simulink model "moto"  (R2026a)
settings: Solver=VariableStepAuto
InitFcn:
  | moto_init;
values from neighbouring files (symbols this model uses):
  nz = [0,0,1].'    [moto_init.m]
  p = motoParameters    [bikeSimToMotoParameters.m]    (also in moto_init.m = bikeSimToPrydeV2Parameters(bs,130/3.6); moto_trim_test.m = P{idx_vx}; steadyTurningTrimEqns.m = in3(41,:); steadyTurningTrimJac.m = in3(41,:))
  Scamber = rscrew('x',p_camber0)    [moto_init.m]
  Spitchr = rscrew('y',p_pitchr0)    [moto_init.m]
  Sx = pscrew('x')    [moto_init.m]
  Sy = pscrew('y')    [moto_init.m]
  Syaw = rscrew('z',p_yaw0)    [moto_init.m]
libraries: simulink_extras x3
settings Model: Creator=marti  LastModifiedBy=marti

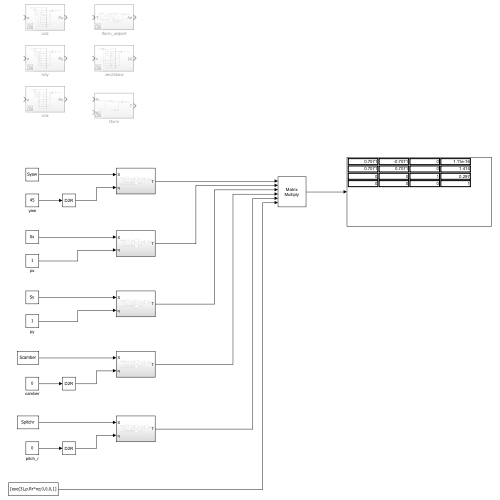
[thumbnail: Simulink's stored preview of the top-level diagram]
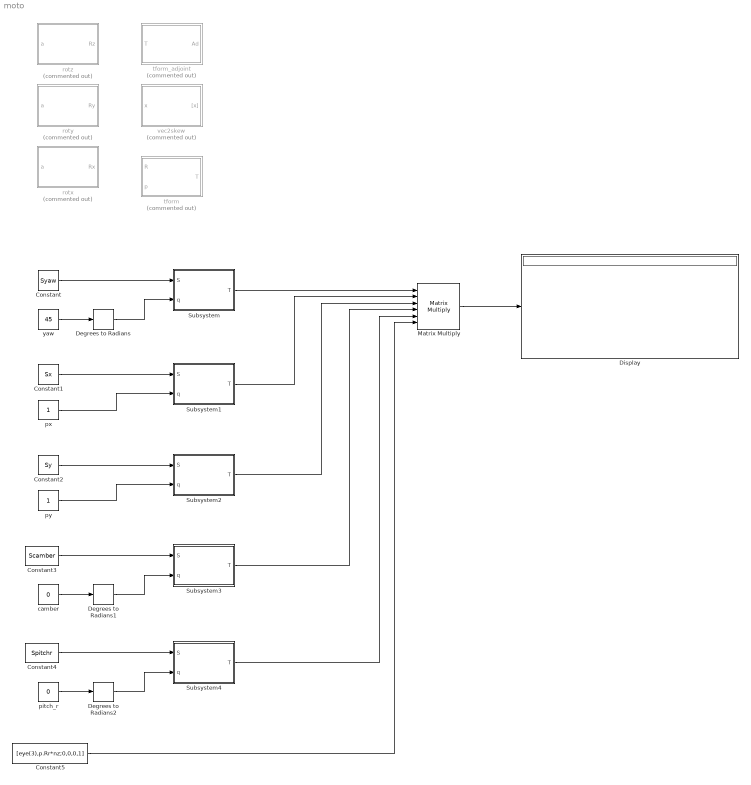
== system moto ==
  Constant : Constant  Value=Syaw
  Constant1 : Constant  Value=Sx
  Constant2 : Constant  Value=Sy
  Constant3 : Constant  Value=Scamber
  Constant4 : Constant  Value=Spitchr
  Constant5 : Constant  Value=[eye(3),p.Rr*nz;0,0,0,1]
  Degrees to Radians : simulink_extras/Transformations/Degrees to Radians
  Degrees to Radians1 : simulink_extras/Transformations/Degrees to Radians
  Degrees to Radians2 : simulink_extras/Transformations/Degrees to Radians
  Display : Display
  Matrix Multiply : Product  Inputs=6  Multiplication=Matrix(*)
  Subsystem : Subsystem
  Subsystem1 : Subsystem
  Subsystem2 : Subsystem
  Subsystem3 : Subsystem
  Subsystem4 : Subsystem
  camber : Constant  Value=0
  pitch_r : Constant  Value=0
  px : Constant
  py : Constant
  rotx : Subsystem  Commented=on
  roty : Subsystem  Commented=on
  rotz : Subsystem  Commented=on
  tform : Subsystem  Commented=on
  tform_adjoint : Subsystem  Commented=on
  vec2skew : Subsystem  Commented=on
  yaw : Constant  Value=45
  wires:
  yaw/1 -> Degrees to Radians/1
  Degrees to Radians/1 -> Subsystem/2(q)
  Constant/1 -> Subsystem/1(S)
  Constant1/1 -> Subsystem1/1(S)
  px/1 -> Subsystem1/2(q)
  Constant2/1 -> Subsystem2/1(S)
  py/1 -> Subsystem2/2(q)
  Constant3/1 -> Subsystem3/1(S)
  Degrees to Radians1/1 -> Subsystem3/2(q)
  camber/1 -> Degrees to Radians1/1
  pitch_r/1 -> Degrees to Radians2/1
  Degrees to Radians2/1 -> Subsystem4/2(q)
  Constant4/1 -> Subsystem4/1(S)
  Subsystem/1(T) -> Matrix Multiply/1
  Subsystem1/1(T) -> Matrix Multiply/2
  Subsystem2/1(T) -> Matrix Multiply/3
  Subsystem3/1(T) -> Matrix Multiply/4
  Subsystem4/1(T) -> Matrix Multiply/5
  Matrix Multiply/1 -> Display/1
  Constant5/1 -> Matrix Multiply/6

== system moto/Subsystem ==
  S : Inport
  q : Inport  Port=2
  Reshape : Reshape  OutputDimensionality=Column vector (2-D)
  Selector : Selector  InputPortWidth=6  IndexOptions=Index vector (dialog)  Indices=1:3  OutputSizes=1
  axisAngleToRotMat : Subsystem
  screwDistanceToPos : Subsystem
  tform : Subsystem
  T : Outport
  wires:
  S/1 -> Reshape/1
  Selector/1 -> axisAngleToRotMat/1(w)  "w"
  q/1 -> screwDistanceToPos/2(q), axisAngleToRotMat/2(q)
  axisAngleToRotMat/1(R) -> tform/1(R)
  tform/1(T) -> T/1
  screwDistanceToPos/1(p) -> tform/2(p)
  Reshape/1 -> screwDistanceToPos/1(S), Selector/1

== system moto/Subsystem1 ==
  S : Inport
  q : Inport  Port=2
  Reshape : Reshape  OutputDimensionality=Column vector (2-D)
  Selector : Selector  InputPortWidth=6  IndexOptions=Index vector (dialog)  Indices=1:3  OutputSizes=1
  axisAngleToRotMat : Subsystem
  screwDistanceToPos : Subsystem
  tform : Subsystem
  T : Outport
  wires:
  S/1 -> Reshape/1
  Selector/1 -> axisAngleToRotMat/1(w)  "w"
  q/1 -> screwDistanceToPos/2(q), axisAngleToRotMat/2(q)
  axisAngleToRotMat/1(R) -> tform/1(R)
  tform/1(T) -> T/1
  screwDistanceToPos/1(p) -> tform/2(p)
  Reshape/1 -> screwDistanceToPos/1(S), Selector/1

== system moto/Subsystem2 ==
  S : Inport
  q : Inport  Port=2
  Reshape : Reshape  OutputDimensionality=Column vector (2-D)
  Selector : Selector  InputPortWidth=6  IndexOptions=Index vector (dialog)  Indices=1:3  OutputSizes=1
  axisAngleToRotMat : Subsystem
  screwDistanceToPos : Subsystem
  tform : Subsystem
  T : Outport
  wires:
  S/1 -> Reshape/1
  Selector/1 -> axisAngleToRotMat/1(w)  "w"
  q/1 -> screwDistanceToPos/2(q), axisAngleToRotMat/2(q)
  axisAngleToRotMat/1(R) -> tform/1(R)
  tform/1(T) -> T/1
  screwDistanceToPos/1(p) -> tform/2(p)
  Reshape/1 -> screwDistanceToPos/1(S), Selector/1

== system moto/Subsystem3 ==
  S : Inport
  q : Inport  Port=2
  Reshape : Reshape  OutputDimensionality=Column vector (2-D)
  Selector : Selector  InputPortWidth=6  IndexOptions=Index vector (dialog)  Indices=1:3  OutputSizes=1
  axisAngleToRotMat : Subsystem
  screwDistanceToPos : Subsystem
  tform : Subsystem
  T : Outport
  wires:
  S/1 -> Reshape/1
  Selector/1 -> axisAngleToRotMat/1(w)  "w"
  q/1 -> screwDistanceToPos/2(q), axisAngleToRotMat/2(q)
  axisAngleToRotMat/1(R) -> tform/1(R)
  tform/1(T) -> T/1
  screwDistanceToPos/1(p) -> tform/2(p)
  Reshape/1 -> screwDistanceToPos/1(S), Selector/1

== system moto/Subsystem4 ==
  S : Inport
  q : Inport  Port=2
  Reshape : Reshape  OutputDimensionality=Column vector (2-D)
  Selector : Selector  InputPortWidth=6  IndexOptions=Index vector (dialog)  Indices=1:3  OutputSizes=1
  axisAngleToRotMat : Subsystem
  screwDistanceToPos : Subsystem
  tform : Subsystem
  T : Outport
  wires:
  S/1 -> Reshape/1
  Selector/1 -> axisAngleToRotMat/1(w)  "w"
  q/1 -> screwDistanceToPos/2(q), axisAngleToRotMat/2(q)
  axisAngleToRotMat/1(R) -> tform/1(R)
  tform/1(T) -> T/1
  screwDistanceToPos/1(p) -> tform/2(p)
  Reshape/1 -> screwDistanceToPos/1(S), Selector/1

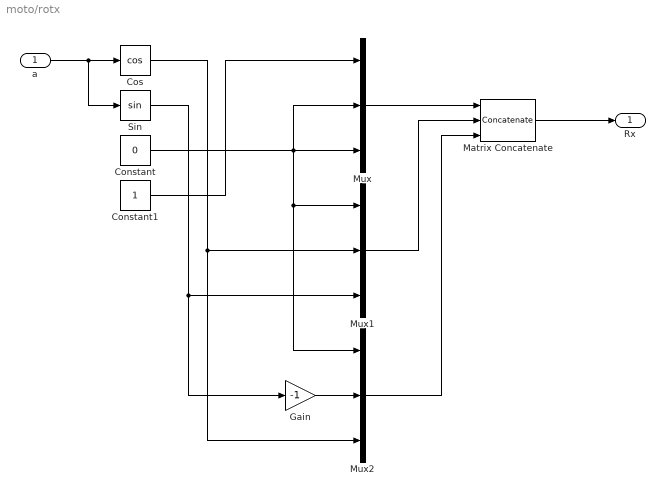
== system moto/rotx ==
  a : Inport
  Constant : Constant  Value=0
  Constant1 : Constant
  Cos : Trigonometry  Operator=cos
  Gain : Gain  Gain=-1
  Matrix Concatenate : Concatenate  NumInputs=3  Mode=Multidimensional array  ConcatenateDimension=2
  Mux : Mux  Inputs=3
  Mux1 : Mux  Inputs=3
  Mux2 : Mux  Inputs=3
  Sin : Trigonometry
  Rx : Outport
  wires:
  a/1 -> Sin/1, Cos/1
  Mux1/1 -> Matrix Concatenate/2
  Mux/1 -> Matrix Concatenate/1
  Mux2/1 -> Matrix Concatenate/3
  Matrix Concatenate/1 -> Rx/1
  Constant1/1 -> Mux/1
  Constant/1 -> Mux2/1, Mux1/1, Mux/3, Mux/2
  Gain/1 -> Mux2/2
  Sin/1 -> Mux1/3, Gain/1
  Cos/1 -> Mux2/3, Mux1/2

== system moto/roty ==
  a : Inport
  Constant : Constant  Value=0
  Constant1 : Constant
  Cos : Trigonometry  Operator=cos
  Gain : Gain  Gain=-1
  Matrix Concatenate : Concatenate  NumInputs=3  Mode=Multidimensional array  ConcatenateDimension=2
  Mux : Mux  Inputs=3
  Mux1 : Mux  Inputs=3
  Mux2 : Mux  Inputs=3
  Sin : Trigonometry
  Ry : Outport
  wires:
  a/1 -> Sin/1, Cos/1
  Mux1/1 -> Matrix Concatenate/2
  Mux/1 -> Matrix Concatenate/1
  Mux2/1 -> Matrix Concatenate/3
  Matrix Concatenate/1 -> Ry/1
  Gain/1 -> Mux/3
  Sin/1 -> Mux2/1, Gain/1
  Cos/1 -> Mux2/3, Mux/1
  Constant/1 -> Mux2/2, Mux1/3, Mux1/1, Mux/2
  Constant1/1 -> Mux1/2

== system moto/rotz ==
  a : Inport
  Constant : Constant  Value=0
  Constant1 : Constant
  Cos : Trigonometry  Operator=cos
  Gain : Gain  Gain=-1
  Matrix Concatenate : Concatenate  NumInputs=3  Mode=Multidimensional array  ConcatenateDimension=2
  Mux : Mux  Inputs=3
  Mux1 : Mux  Inputs=3
  Mux2 : Mux  Inputs=3
  Sin : Trigonometry
  Rz : Outport
  wires:
  Cos/1 -> Mux1/2, Mux/1
  Constant1/1 -> Mux2/3
  Sin/1 -> Mux/2, Gain/1
  a/1 -> Sin/1, Cos/1
  Constant/1 -> Mux/3, Mux2/2, Mux2/1, Mux1/3
  Gain/1 -> Mux1/1
  Mux1/1 -> Matrix Concatenate/2
  Mux/1 -> Matrix Concatenate/1
  Mux2/1 -> Matrix Concatenate/3
  Matrix Concatenate/1 -> Rz/1

== system moto/tform ==
  R : Inport
  p : Inport  Port=2
  Constant : Constant  Value=[0,0,0,1]
  Matrix Concatenate : Concatenate  Mode=Multidimensional array  ConcatenateDimension=2
  Matrix Concatenate2 : Concatenate  Mode=Multidimensional array
  Reshape : Reshape  OutputDimensionality=Row vector (2-D)
  T : Outport
  wires:
  p/1 -> Matrix Concatenate/2
  Constant/1 -> Reshape/1
  Matrix Concatenate/1 -> Matrix Concatenate2/1
  Matrix Concatenate2/1 -> T/1
  R/1 -> Matrix Concatenate/1
  Reshape/1 -> Matrix Concatenate2/2

== system moto/tform_adjoint ==
  T : Inport
  Constant : Constant  Value=zeros(3)
  Matrix Concatenate : Concatenate  Mode=Multidimensional array  ConcatenateDimension=2
  Matrix Concatenate1 : Concatenate  Mode=Multidimensional array  ConcatenateDimension=2
  Matrix Concatenate2 : Concatenate  Mode=Multidimensional array
  Matrix Multiply : Product  Multiplication=Matrix(*)
  Selector : Selector  NumberOfDimensions=2  InputPortWidth=3  IndexOptions=Index vector (dialog),Index vector (dialog)  Indices=1:3,1:3  OutputSizes=1,1
  Selector1 : Selector  NumberOfDimensions=2  InputPortWidth=3  IndexOptions=Index vector (dialog),Index vector (dialog)  Indices=1:3,4  OutputSizes=1,1
  vec2skew : Subsystem
  Ad : Outport
  wires:
  Selector1/1 -> vec2skew/1(x)
  Selector/1 -> Matrix Multiply/2, Matrix Concatenate1/2, Matrix Concatenate/1
  Constant/1 -> Matrix Concatenate/2
  vec2skew/1("[x]") -> Matrix Multiply/1
  Matrix Multiply/1 -> Matrix Concatenate1/1
  Matrix Concatenate1/1 -> Matrix Concatenate2/2
  Matrix Concatenate/1 -> Matrix Concatenate2/1
  Matrix Concatenate2/1 -> Ad/1
  T/1 -> Selector1/1, Selector/1

== system moto/vec2skew ==
  x : Inport
  Constant : Constant  Value=0
  Demux : Demux  Outputs=3
  Gain : Gain  Gain=-1
  Gain1 : Gain  Gain=-1
  Gain2 : Gain  Gain=-1
  Matrix Concatenate : Concatenate  NumInputs=3  Mode=Multidimensional array  ConcatenateDimension=2
  Mux : Mux  Inputs=3
  Mux1 : Mux  Inputs=3
  Mux2 : Mux  Inputs=3
  "[x]" : Outport
  wires:
  Mux1/1 -> Matrix Concatenate/2
  Mux/1 -> Matrix Concatenate/1
  Mux2/1 -> Matrix Concatenate/3
  Matrix Concatenate/1 -> "[x]"/1
  Gain/1 -> Mux/3
  Gain1/1 -> Mux1/1
  Gain2/1 -> Mux2/2
  Constant/1 -> Mux/1, Mux1/2, Mux2/3
  x/1 -> Demux/1
  Demux/3 -> Gain1/1, Mux/2  "z"
  Demux/2 -> Mux2/1, Gain/1  "y"
  Demux/1 -> Gain2/1, Mux1/3  "x"

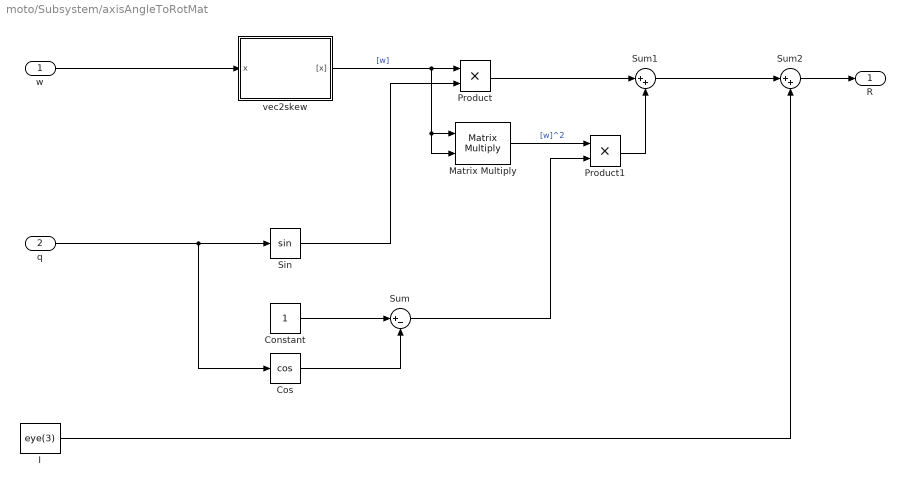
== system moto/Subsystem/axisAngleToRotMat ==
  w : Inport
  q : Inport  Port=2
  Constant : Constant
  Cos : Trigonometry  Operator=cos
  I : Constant  Value=eye(3)
  Matrix Multiply : Product  Multiplication=Matrix(*)
  Product : Product
  Product1 : Product
  Sin : Trigonometry
  Sum : Sum  Inputs=|+-
  Sum1 : Sum  Inputs=|++
  Sum2 : Sum  Inputs=|++
  vec2skew : Subsystem
  R : Outport
  wires:
  Cos/1 -> Sum/2
  Sum1/1 -> Sum2/1
  Sum/1 -> Product1/2
  Matrix Multiply/1 -> Product1/1  "[w]^2"
  Product1/1 -> Sum1/2
  Constant/1 -> Sum/1
  Product/1 -> Sum1/1
  I/1 -> Sum2/2
  vec2skew/1("[x]") -> Matrix Multiply/2, Matrix Multiply/1, Product/1  "[w]"
  Sin/1 -> Product/2
  q/1 -> Cos/1, Sin/1
  Sum2/1 -> R/1
  w/1 -> vec2skew/1(x)

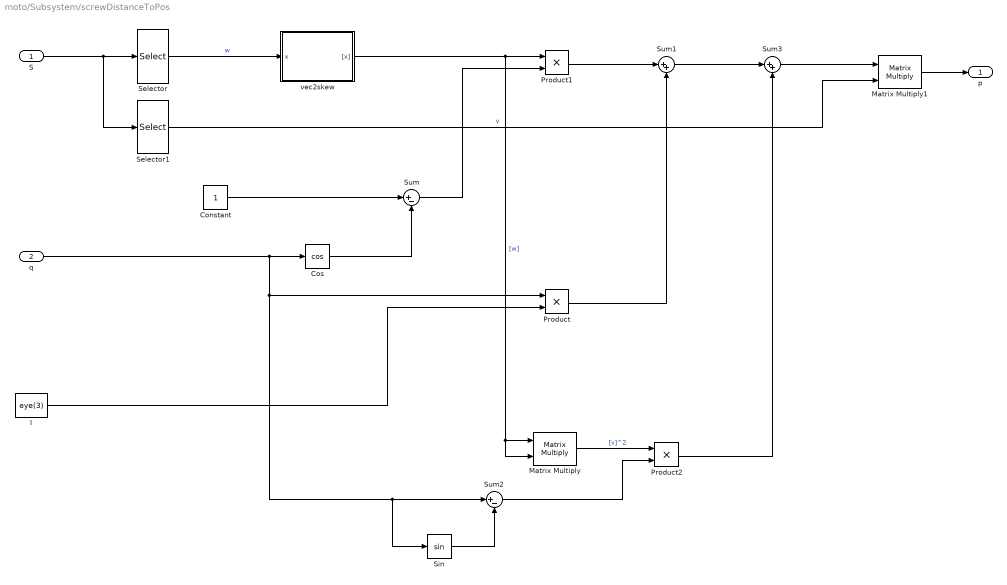
== system moto/Subsystem/screwDistanceToPos ==
  S : Inport
  q : Inport  Port=2
  Constant : Constant
  Cos : Trigonometry  Operator=cos
  I : Constant  Value=eye(3)
  Matrix Multiply : Product  Multiplication=Matrix(*)
  Matrix Multiply1 : Product  Multiplication=Matrix(*)
  Product : Product
  Product1 : Product
  Product2 : Product
  Selector : Selector  InputPortWidth=6  IndexOptions=Index vector (dialog)  Indices=1:3  OutputSizes=1
  Selector1 : Selector  InputPortWidth=6  IndexOptions=Index vector (dialog)  Indices=4:6  OutputSizes=1
  Sin : Trigonometry
  Sum : Sum  Inputs=|+-
  Sum1 : Sum  Inputs=|++
  Sum2 : Sum  Inputs=|+-
  Sum3 : Sum  Inputs=|++
  vec2skew : Subsystem
  p : Outport
  wires:
  Product/1 -> Sum1/2
  q/1 -> Cos/1, Product/1, Sin/1, Sum2/1
  Cos/1 -> Sum/2
  Constant/1 -> Sum/1
  vec2skew/1("[x]") -> Matrix Multiply/2, Matrix Multiply/1, Product1/1  "[w]"
  Sum2/1 -> Product2/2
  I/1 -> Product/2
  Product1/1 -> Sum1/1
  Sum/1 -> Product1/2
  Matrix Multiply/1 -> Product2/1  "[v]^2"
  Sum3/1 -> Matrix Multiply1/1
  Product2/1 -> Sum3/2
  Sin/1 -> Sum2/2
  Sum1/1 -> Sum3/1
  Selector1/1 -> Matrix Multiply1/2  "v"
  Matrix Multiply1/1 -> p/1
  Selector/1 -> vec2skew/1(x)  "w"
  S/1 -> Selector1/1, Selector/1

== system moto/Subsystem/tform ==
  R : Inport
  p : Inport  Port=2
  Constant : Constant  Value=[0,0,0,1]
  Matrix Concatenate : Concatenate  Mode=Multidimensional array  ConcatenateDimension=2
  Matrix Concatenate2 : Concatenate  Mode=Multidimensional array
  Reshape : Reshape  OutputDimensionality=Row vector (2-D)
  T : Outport
  wires:
  p/1 -> Matrix Concatenate/2
  Constant/1 -> Reshape/1
  Matrix Concatenate/1 -> Matrix Concatenate2/1
  Matrix Concatenate2/1 -> T/1
  R/1 -> Matrix Concatenate/1
  Reshape/1 -> Matrix Concatenate2/2

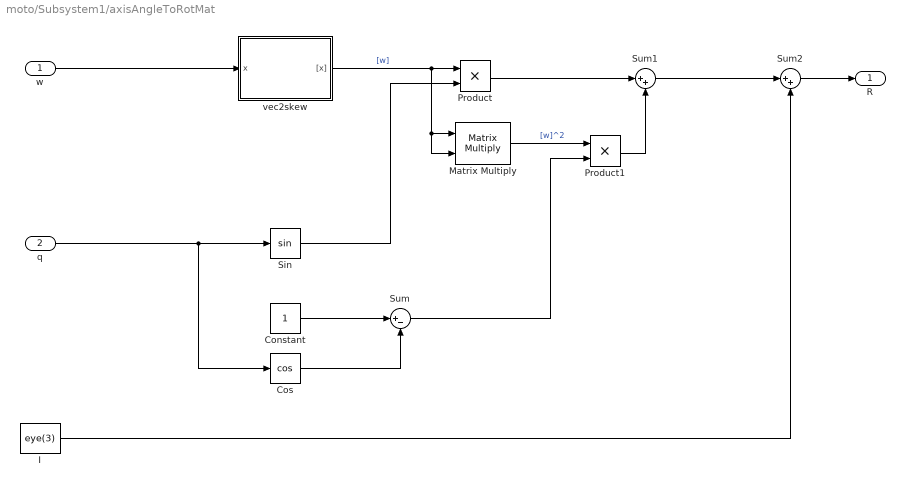
== system moto/Subsystem1/axisAngleToRotMat ==
  w : Inport
  q : Inport  Port=2
  Constant : Constant
  Cos : Trigonometry  Operator=cos
  I : Constant  Value=eye(3)
  Matrix Multiply : Product  Multiplication=Matrix(*)
  Product : Product
  Product1 : Product
  Sin : Trigonometry
  Sum : Sum  Inputs=|+-
  Sum1 : Sum  Inputs=|++
  Sum2 : Sum  Inputs=|++
  vec2skew : Subsystem
  R : Outport
  wires:
  Cos/1 -> Sum/2
  Sum1/1 -> Sum2/1
  Sum/1 -> Product1/2
  Matrix Multiply/1 -> Product1/1  "[w]^2"
  Product1/1 -> Sum1/2
  Constant/1 -> Sum/1
  Product/1 -> Sum1/1
  I/1 -> Sum2/2
  vec2skew/1("[x]") -> Matrix Multiply/2, Matrix Multiply/1, Product/1  "[w]"
  Sin/1 -> Product/2
  q/1 -> Cos/1, Sin/1
  Sum2/1 -> R/1
  w/1 -> vec2skew/1(x)

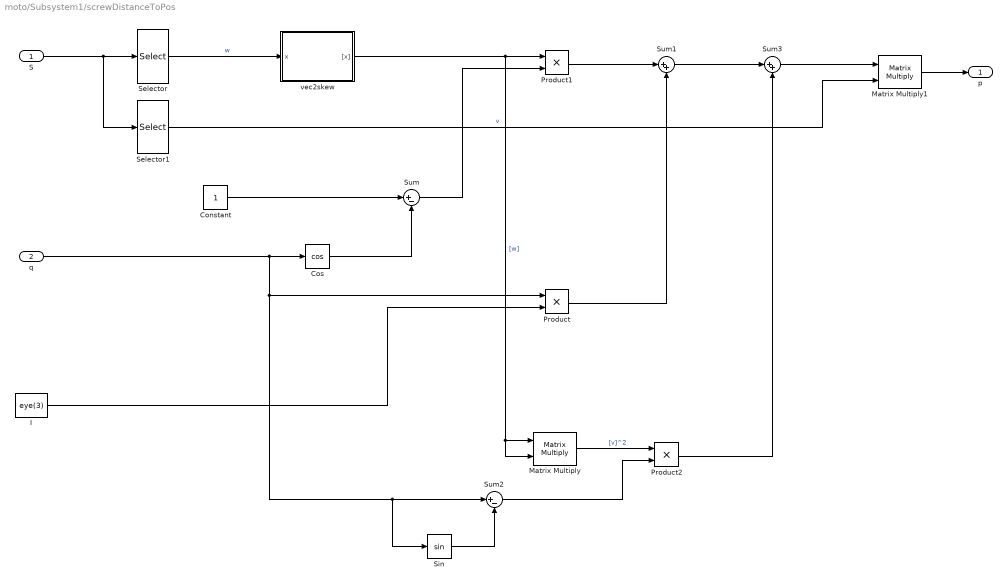
== system moto/Subsystem1/screwDistanceToPos ==
  S : Inport
  q : Inport  Port=2
  Constant : Constant
  Cos : Trigonometry  Operator=cos
  I : Constant  Value=eye(3)
  Matrix Multiply : Product  Multiplication=Matrix(*)
  Matrix Multiply1 : Product  Multiplication=Matrix(*)
  Product : Product
  Product1 : Product
  Product2 : Product
  Selector : Selector  InputPortWidth=6  IndexOptions=Index vector (dialog)  Indices=1:3  OutputSizes=1
  Selector1 : Selector  InputPortWidth=6  IndexOptions=Index vector (dialog)  Indices=4:6  OutputSizes=1
  Sin : Trigonometry
  Sum : Sum  Inputs=|+-
  Sum1 : Sum  Inputs=|++
  Sum2 : Sum  Inputs=|+-
  Sum3 : Sum  Inputs=|++
  vec2skew : Subsystem
  p : Outport
  wires:
  Product/1 -> Sum1/2
  q/1 -> Cos/1, Product/1, Sin/1, Sum2/1
  Cos/1 -> Sum/2
  Constant/1 -> Sum/1
  vec2skew/1("[x]") -> Matrix Multiply/2, Matrix Multiply/1, Product1/1  "[w]"
  Sum2/1 -> Product2/2
  I/1 -> Product/2
  Product1/1 -> Sum1/1
  Sum/1 -> Product1/2
  Matrix Multiply/1 -> Product2/1  "[v]^2"
  Sum3/1 -> Matrix Multiply1/1
  Product2/1 -> Sum3/2
  Sin/1 -> Sum2/2
  Sum1/1 -> Sum3/1
  Selector1/1 -> Matrix Multiply1/2  "v"
  Matrix Multiply1/1 -> p/1
  Selector/1 -> vec2skew/1(x)  "w"
  S/1 -> Selector1/1, Selector/1

== system moto/Subsystem1/tform ==
  R : Inport
  p : Inport  Port=2
  Constant : Constant  Value=[0,0,0,1]
  Matrix Concatenate : Concatenate  Mode=Multidimensional array  ConcatenateDimension=2
  Matrix Concatenate2 : Concatenate  Mode=Multidimensional array
  Reshape : Reshape  OutputDimensionality=Row vector (2-D)
  T : Outport
  wires:
  p/1 -> Matrix Concatenate/2
  Constant/1 -> Reshape/1
  Matrix Concatenate/1 -> Matrix Concatenate2/1
  Matrix Concatenate2/1 -> T/1
  R/1 -> Matrix Concatenate/1
  Reshape/1 -> Matrix Concatenate2/2

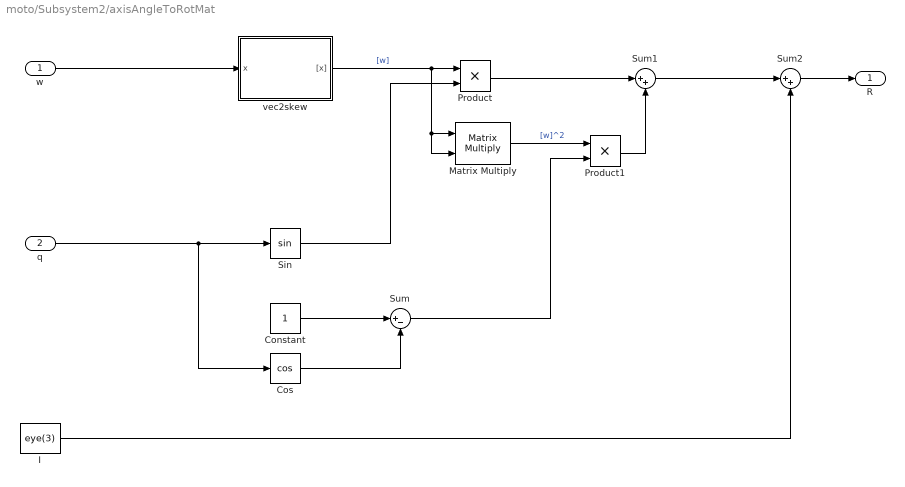
== system moto/Subsystem2/axisAngleToRotMat ==
  w : Inport
  q : Inport  Port=2
  Constant : Constant
  Cos : Trigonometry  Operator=cos
  I : Constant  Value=eye(3)
  Matrix Multiply : Product  Multiplication=Matrix(*)
  Product : Product
  Product1 : Product
  Sin : Trigonometry
  Sum : Sum  Inputs=|+-
  Sum1 : Sum  Inputs=|++
  Sum2 : Sum  Inputs=|++
  vec2skew : Subsystem
  R : Outport
  wires:
  Cos/1 -> Sum/2
  Sum1/1 -> Sum2/1
  Sum/1 -> Product1/2
  Matrix Multiply/1 -> Product1/1  "[w]^2"
  Product1/1 -> Sum1/2
  Constant/1 -> Sum/1
  Product/1 -> Sum1/1
  I/1 -> Sum2/2
  vec2skew/1("[x]") -> Matrix Multiply/2, Matrix Multiply/1, Product/1  "[w]"
  Sin/1 -> Product/2
  q/1 -> Cos/1, Sin/1
  Sum2/1 -> R/1
  w/1 -> vec2skew/1(x)

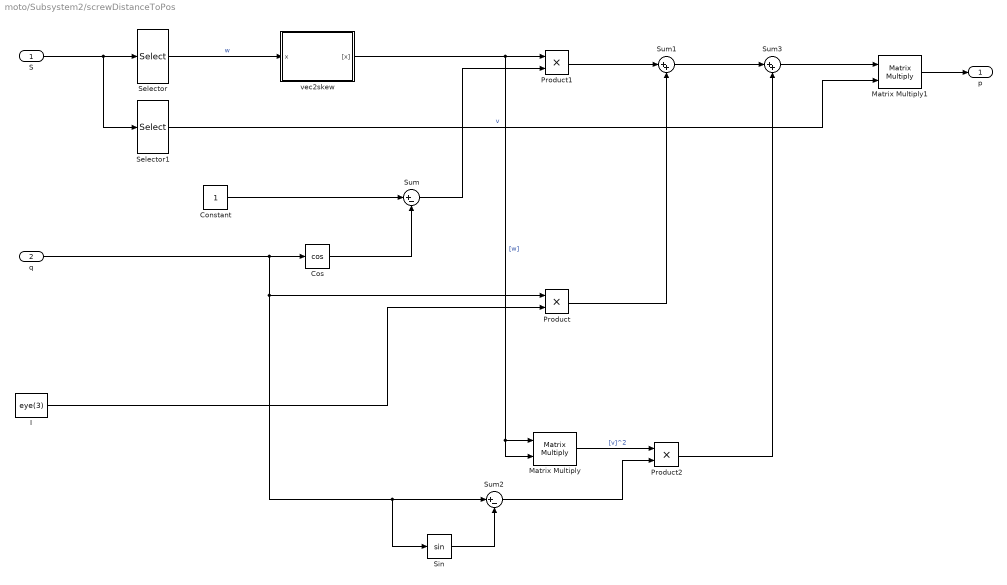
== system moto/Subsystem2/screwDistanceToPos ==
  S : Inport
  q : Inport  Port=2
  Constant : Constant
  Cos : Trigonometry  Operator=cos
  I : Constant  Value=eye(3)
  Matrix Multiply : Product  Multiplication=Matrix(*)
  Matrix Multiply1 : Product  Multiplication=Matrix(*)
  Product : Product
  Product1 : Product
  Product2 : Product
  Selector : Selector  InputPortWidth=6  IndexOptions=Index vector (dialog)  Indices=1:3  OutputSizes=1
  Selector1 : Selector  InputPortWidth=6  IndexOptions=Index vector (dialog)  Indices=4:6  OutputSizes=1
  Sin : Trigonometry
  Sum : Sum  Inputs=|+-
  Sum1 : Sum  Inputs=|++
  Sum2 : Sum  Inputs=|+-
  Sum3 : Sum  Inputs=|++
  vec2skew : Subsystem
  p : Outport
  wires:
  Product/1 -> Sum1/2
  q/1 -> Cos/1, Product/1, Sin/1, Sum2/1
  Cos/1 -> Sum/2
  Constant/1 -> Sum/1
  vec2skew/1("[x]") -> Matrix Multiply/2, Matrix Multiply/1, Product1/1  "[w]"
  Sum2/1 -> Product2/2
  I/1 -> Product/2
  Product1/1 -> Sum1/1
  Sum/1 -> Product1/2
  Matrix Multiply/1 -> Product2/1  "[v]^2"
  Sum3/1 -> Matrix Multiply1/1
  Product2/1 -> Sum3/2
  Sin/1 -> Sum2/2
  Sum1/1 -> Sum3/1
  Selector1/1 -> Matrix Multiply1/2  "v"
  Matrix Multiply1/1 -> p/1
  Selector/1 -> vec2skew/1(x)  "w"
  S/1 -> Selector1/1, Selector/1

== system moto/Subsystem2/tform ==
  R : Inport
  p : Inport  Port=2
  Constant : Constant  Value=[0,0,0,1]
  Matrix Concatenate : Concatenate  Mode=Multidimensional array  ConcatenateDimension=2
  Matrix Concatenate2 : Concatenate  Mode=Multidimensional array
  Reshape : Reshape  OutputDimensionality=Row vector (2-D)
  T : Outport
  wires:
  p/1 -> Matrix Concatenate/2
  Constant/1 -> Reshape/1
  Matrix Concatenate/1 -> Matrix Concatenate2/1
  Matrix Concatenate2/1 -> T/1
  R/1 -> Matrix Concatenate/1
  Reshape/1 -> Matrix Concatenate2/2

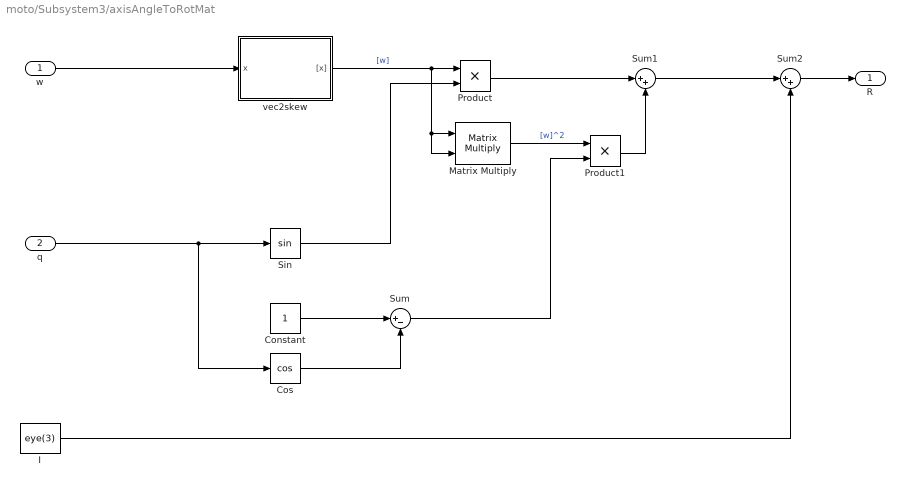
== system moto/Subsystem3/axisAngleToRotMat ==
  w : Inport
  q : Inport  Port=2
  Constant : Constant
  Cos : Trigonometry  Operator=cos
  I : Constant  Value=eye(3)
  Matrix Multiply : Product  Multiplication=Matrix(*)
  Product : Product
  Product1 : Product
  Sin : Trigonometry
  Sum : Sum  Inputs=|+-
  Sum1 : Sum  Inputs=|++
  Sum2 : Sum  Inputs=|++
  vec2skew : Subsystem
  R : Outport
  wires:
  Cos/1 -> Sum/2
  Sum1/1 -> Sum2/1
  Sum/1 -> Product1/2
  Matrix Multiply/1 -> Product1/1  "[w]^2"
  Product1/1 -> Sum1/2
  Constant/1 -> Sum/1
  Product/1 -> Sum1/1
  I/1 -> Sum2/2
  vec2skew/1("[x]") -> Matrix Multiply/2, Matrix Multiply/1, Product/1  "[w]"
  Sin/1 -> Product/2
  q/1 -> Cos/1, Sin/1
  Sum2/1 -> R/1
  w/1 -> vec2skew/1(x)

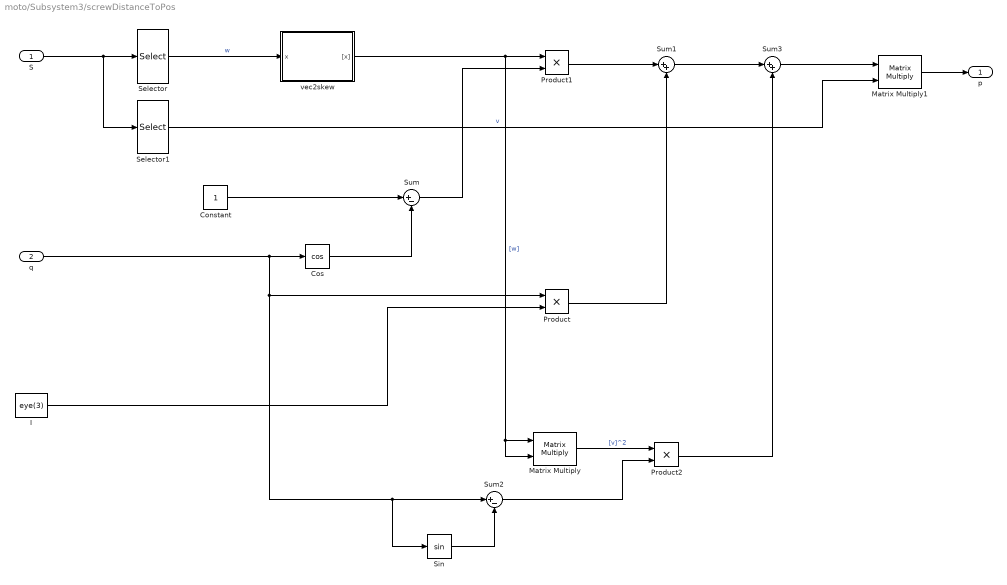
== system moto/Subsystem3/screwDistanceToPos ==
  S : Inport
  q : Inport  Port=2
  Constant : Constant
  Cos : Trigonometry  Operator=cos
  I : Constant  Value=eye(3)
  Matrix Multiply : Product  Multiplication=Matrix(*)
  Matrix Multiply1 : Product  Multiplication=Matrix(*)
  Product : Product
  Product1 : Product
  Product2 : Product
  Selector : Selector  InputPortWidth=6  IndexOptions=Index vector (dialog)  Indices=1:3  OutputSizes=1
  Selector1 : Selector  InputPortWidth=6  IndexOptions=Index vector (dialog)  Indices=4:6  OutputSizes=1
  Sin : Trigonometry
  Sum : Sum  Inputs=|+-
  Sum1 : Sum  Inputs=|++
  Sum2 : Sum  Inputs=|+-
  Sum3 : Sum  Inputs=|++
  vec2skew : Subsystem
  p : Outport
  wires:
  Product/1 -> Sum1/2
  q/1 -> Cos/1, Product/1, Sin/1, Sum2/1
  Cos/1 -> Sum/2
  Constant/1 -> Sum/1
  vec2skew/1("[x]") -> Matrix Multiply/2, Matrix Multiply/1, Product1/1  "[w]"
  Sum2/1 -> Product2/2
  I/1 -> Product/2
  Product1/1 -> Sum1/1
  Sum/1 -> Product1/2
  Matrix Multiply/1 -> Product2/1  "[v]^2"
  Sum3/1 -> Matrix Multiply1/1
  Product2/1 -> Sum3/2
  Sin/1 -> Sum2/2
  Sum1/1 -> Sum3/1
  Selector1/1 -> Matrix Multiply1/2  "v"
  Matrix Multiply1/1 -> p/1
  Selector/1 -> vec2skew/1(x)  "w"
  S/1 -> Selector1/1, Selector/1

== system moto/Subsystem3/tform ==
  R : Inport
  p : Inport  Port=2
  Constant : Constant  Value=[0,0,0,1]
  Matrix Concatenate : Concatenate  Mode=Multidimensional array  ConcatenateDimension=2
  Matrix Concatenate2 : Concatenate  Mode=Multidimensional array
  Reshape : Reshape  OutputDimensionality=Row vector (2-D)
  T : Outport
  wires:
  p/1 -> Matrix Concatenate/2
  Constant/1 -> Reshape/1
  Matrix Concatenate/1 -> Matrix Concatenate2/1
  Matrix Concatenate2/1 -> T/1
  R/1 -> Matrix Concatenate/1
  Reshape/1 -> Matrix Concatenate2/2

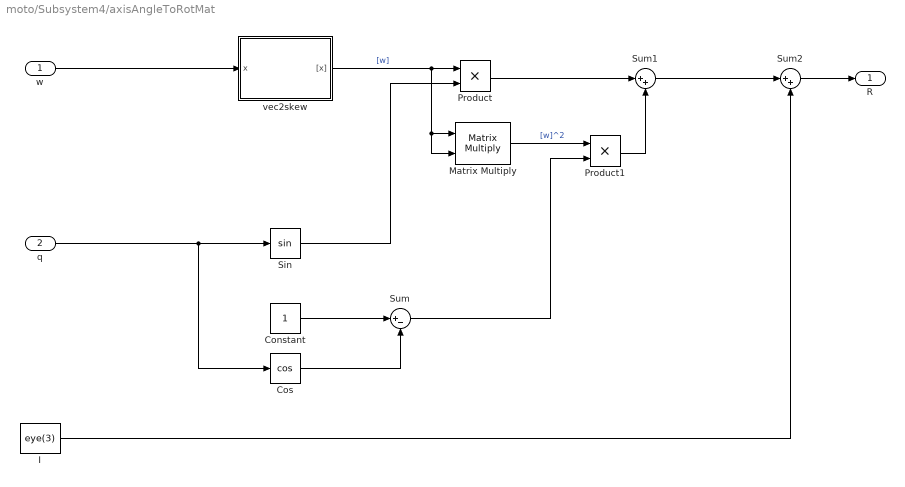
== system moto/Subsystem4/axisAngleToRotMat ==
  w : Inport
  q : Inport  Port=2
  Constant : Constant
  Cos : Trigonometry  Operator=cos
  I : Constant  Value=eye(3)
  Matrix Multiply : Product  Multiplication=Matrix(*)
  Product : Product
  Product1 : Product
  Sin : Trigonometry
  Sum : Sum  Inputs=|+-
  Sum1 : Sum  Inputs=|++
  Sum2 : Sum  Inputs=|++
  vec2skew : Subsystem
  R : Outport
  wires:
  Cos/1 -> Sum/2
  Sum1/1 -> Sum2/1
  Sum/1 -> Product1/2
  Matrix Multiply/1 -> Product1/1  "[w]^2"
  Product1/1 -> Sum1/2
  Constant/1 -> Sum/1
  Product/1 -> Sum1/1
  I/1 -> Sum2/2
  vec2skew/1("[x]") -> Matrix Multiply/2, Matrix Multiply/1, Product/1  "[w]"
  Sin/1 -> Product/2
  q/1 -> Cos/1, Sin/1
  Sum2/1 -> R/1
  w/1 -> vec2skew/1(x)

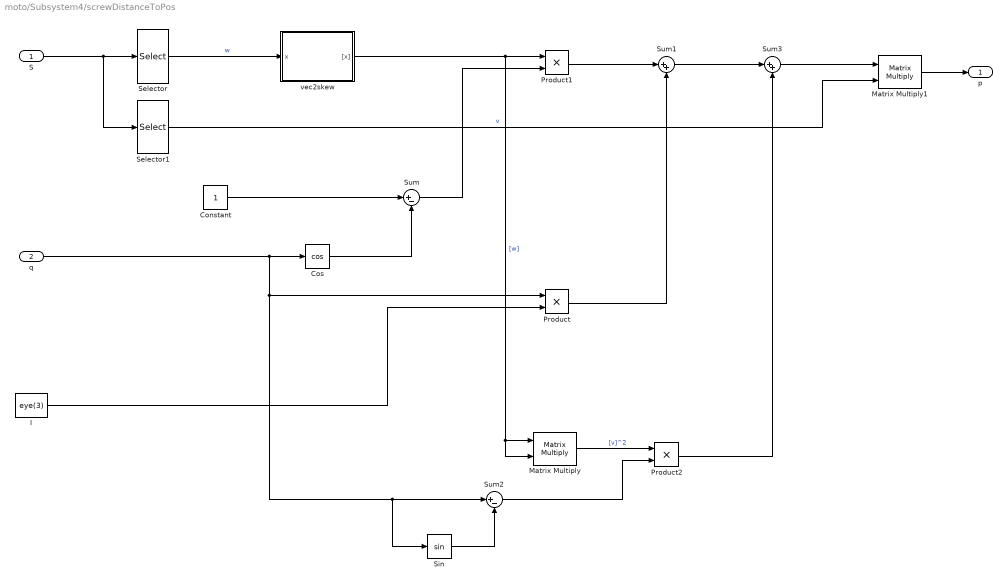
== system moto/Subsystem4/screwDistanceToPos ==
  S : Inport
  q : Inport  Port=2
  Constant : Constant
  Cos : Trigonometry  Operator=cos
  I : Constant  Value=eye(3)
  Matrix Multiply : Product  Multiplication=Matrix(*)
  Matrix Multiply1 : Product  Multiplication=Matrix(*)
  Product : Product
  Product1 : Product
  Product2 : Product
  Selector : Selector  InputPortWidth=6  IndexOptions=Index vector (dialog)  Indices=1:3  OutputSizes=1
  Selector1 : Selector  InputPortWidth=6  IndexOptions=Index vector (dialog)  Indices=4:6  OutputSizes=1
  Sin : Trigonometry
  Sum : Sum  Inputs=|+-
  Sum1 : Sum  Inputs=|++
  Sum2 : Sum  Inputs=|+-
  Sum3 : Sum  Inputs=|++
  vec2skew : Subsystem
  p : Outport
  wires:
  Product/1 -> Sum1/2
  q/1 -> Cos/1, Product/1, Sin/1, Sum2/1
  Cos/1 -> Sum/2
  Constant/1 -> Sum/1
  vec2skew/1("[x]") -> Matrix Multiply/2, Matrix Multiply/1, Product1/1  "[w]"
  Sum2/1 -> Product2/2
  I/1 -> Product/2
  Product1/1 -> Sum1/1
  Sum/1 -> Product1/2
  Matrix Multiply/1 -> Product2/1  "[v]^2"
  Sum3/1 -> Matrix Multiply1/1
  Product2/1 -> Sum3/2
  Sin/1 -> Sum2/2
  Sum1/1 -> Sum3/1
  Selector1/1 -> Matrix Multiply1/2  "v"
  Matrix Multiply1/1 -> p/1
  Selector/1 -> vec2skew/1(x)  "w"
  S/1 -> Selector1/1, Selector/1

== system moto/Subsystem4/tform ==
  R : Inport
  p : Inport  Port=2
  Constant : Constant  Value=[0,0,0,1]
  Matrix Concatenate : Concatenate  Mode=Multidimensional array  ConcatenateDimension=2
  Matrix Concatenate2 : Concatenate  Mode=Multidimensional array
  Reshape : Reshape  OutputDimensionality=Row vector (2-D)
  T : Outport
  wires:
  p/1 -> Matrix Concatenate/2
  Constant/1 -> Reshape/1
  Matrix Concatenate/1 -> Matrix Concatenate2/1
  Matrix Concatenate2/1 -> T/1
  R/1 -> Matrix Concatenate/1
  Reshape/1 -> Matrix Concatenate2/2

== system moto/tform_adjoint/vec2skew ==
  x : Inport
  Constant : Constant  Value=0
  Demux : Demux  Outputs=3
  Gain : Gain  Gain=-1
  Gain1 : Gain  Gain=-1
  Gain2 : Gain  Gain=-1
  Matrix Concatenate : Concatenate  NumInputs=3  Mode=Multidimensional array  ConcatenateDimension=2
  Mux : Mux  Inputs=3
  Mux1 : Mux  Inputs=3
  Mux2 : Mux  Inputs=3
  "[x]" : Outport
  wires:
  Mux1/1 -> Matrix Concatenate/2
  Mux/1 -> Matrix Concatenate/1
  Mux2/1 -> Matrix Concatenate/3
  Matrix Concatenate/1 -> "[x]"/1
  Gain/1 -> Mux/3
  Gain1/1 -> Mux1/1
  Gain2/1 -> Mux2/2
  Constant/1 -> Mux/1, Mux1/2, Mux2/3
  x/1 -> Demux/1
  Demux/3 -> Gain1/1, Mux/2  "z"
  Demux/2 -> Mux2/1, Gain/1  "y"
  Demux/1 -> Gain2/1, Mux1/3  "x"

== system moto/Subsystem/axisAngleToRotMat/vec2skew ==
  x : Inport
  Constant : Constant  Value=0
  Demux : Demux  Outputs=3
  Gain : Gain  Gain=-1
  Gain1 : Gain  Gain=-1
  Gain2 : Gain  Gain=-1
  Matrix Concatenate : Concatenate  NumInputs=3  Mode=Multidimensional array  ConcatenateDimension=2
  Mux : Mux  Inputs=3
  Mux1 : Mux  Inputs=3
  Mux2 : Mux  Inputs=3
  "[x]" : Outport
  wires:
  Mux1/1 -> Matrix Concatenate/2
  Mux/1 -> Matrix Concatenate/1
  Mux2/1 -> Matrix Concatenate/3
  Matrix Concatenate/1 -> "[x]"/1
  Gain/1 -> Mux/3
  Gain1/1 -> Mux1/1
  Gain2/1 -> Mux2/2
  Constant/1 -> Mux/1, Mux1/2, Mux2/3
  x/1 -> Demux/1
  Demux/3 -> Gain1/1, Mux/2  "z"
  Demux/2 -> Mux2/1, Gain/1  "y"
  Demux/1 -> Gain2/1, Mux1/3  "x"

== system moto/Subsystem/screwDistanceToPos/vec2skew ==
  x : Inport
  Constant : Constant  Value=0
  Demux : Demux  Outputs=3
  Gain : Gain  Gain=-1
  Gain1 : Gain  Gain=-1
  Gain2 : Gain  Gain=-1
  Matrix Concatenate : Concatenate  NumInputs=3  Mode=Multidimensional array  ConcatenateDimension=2
  Mux : Mux  Inputs=3
  Mux1 : Mux  Inputs=3
  Mux2 : Mux  Inputs=3
  "[x]" : Outport
  wires:
  Mux1/1 -> Matrix Concatenate/2
  Mux/1 -> Matrix Concatenate/1
  Mux2/1 -> Matrix Concatenate/3
  Matrix Concatenate/1 -> "[x]"/1
  Gain/1 -> Mux/3
  Gain1/1 -> Mux1/1
  Gain2/1 -> Mux2/2
  Constant/1 -> Mux/1, Mux1/2, Mux2/3
  x/1 -> Demux/1
  Demux/3 -> Gain1/1, Mux/2  "z"
  Demux/2 -> Mux2/1, Gain/1  "y"
  Demux/1 -> Gain2/1, Mux1/3  "x"

== system moto/Subsystem1/axisAngleToRotMat/vec2skew ==
  x : Inport
  Constant : Constant  Value=0
  Demux : Demux  Outputs=3
  Gain : Gain  Gain=-1
  Gain1 : Gain  Gain=-1
  Gain2 : Gain  Gain=-1
  Matrix Concatenate : Concatenate  NumInputs=3  Mode=Multidimensional array  ConcatenateDimension=2
  Mux : Mux  Inputs=3
  Mux1 : Mux  Inputs=3
  Mux2 : Mux  Inputs=3
  "[x]" : Outport
  wires:
  Mux1/1 -> Matrix Concatenate/2
  Mux/1 -> Matrix Concatenate/1
  Mux2/1 -> Matrix Concatenate/3
  Matrix Concatenate/1 -> "[x]"/1
  Gain/1 -> Mux/3
  Gain1/1 -> Mux1/1
  Gain2/1 -> Mux2/2
  Constant/1 -> Mux/1, Mux1/2, Mux2/3
  x/1 -> Demux/1
  Demux/3 -> Gain1/1, Mux/2  "z"
  Demux/2 -> Mux2/1, Gain/1  "y"
  Demux/1 -> Gain2/1, Mux1/3  "x"

== system moto/Subsystem1/screwDistanceToPos/vec2skew ==
  x : Inport
  Constant : Constant  Value=0
  Demux : Demux  Outputs=3
  Gain : Gain  Gain=-1
  Gain1 : Gain  Gain=-1
  Gain2 : Gain  Gain=-1
  Matrix Concatenate : Concatenate  NumInputs=3  Mode=Multidimensional array  ConcatenateDimension=2
  Mux : Mux  Inputs=3
  Mux1 : Mux  Inputs=3
  Mux2 : Mux  Inputs=3
  "[x]" : Outport
  wires:
  Mux1/1 -> Matrix Concatenate/2
  Mux/1 -> Matrix Concatenate/1
  Mux2/1 -> Matrix Concatenate/3
  Matrix Concatenate/1 -> "[x]"/1
  Gain/1 -> Mux/3
  Gain1/1 -> Mux1/1
  Gain2/1 -> Mux2/2
  Constant/1 -> Mux/1, Mux1/2, Mux2/3
  x/1 -> Demux/1
  Demux/3 -> Gain1/1, Mux/2  "z"
  Demux/2 -> Mux2/1, Gain/1  "y"
  Demux/1 -> Gain2/1, Mux1/3  "x"

== system moto/Subsystem2/axisAngleToRotMat/vec2skew ==
  x : Inport
  Constant : Constant  Value=0
  Demux : Demux  Outputs=3
  Gain : Gain  Gain=-1
  Gain1 : Gain  Gain=-1
  Gain2 : Gain  Gain=-1
  Matrix Concatenate : Concatenate  NumInputs=3  Mode=Multidimensional array  ConcatenateDimension=2
  Mux : Mux  Inputs=3
  Mux1 : Mux  Inputs=3
  Mux2 : Mux  Inputs=3
  "[x]" : Outport
  wires:
  Mux1/1 -> Matrix Concatenate/2
  Mux/1 -> Matrix Concatenate/1
  Mux2/1 -> Matrix Concatenate/3
  Matrix Concatenate/1 -> "[x]"/1
  Gain/1 -> Mux/3
  Gain1/1 -> Mux1/1
  Gain2/1 -> Mux2/2
  Constant/1 -> Mux/1, Mux1/2, Mux2/3
  x/1 -> Demux/1
  Demux/3 -> Gain1/1, Mux/2  "z"
  Demux/2 -> Mux2/1, Gain/1  "y"
  Demux/1 -> Gain2/1, Mux1/3  "x"

== system moto/Subsystem2/screwDistanceToPos/vec2skew ==
  x : Inport
  Constant : Constant  Value=0
  Demux : Demux  Outputs=3
  Gain : Gain  Gain=-1
  Gain1 : Gain  Gain=-1
  Gain2 : Gain  Gain=-1
  Matrix Concatenate : Concatenate  NumInputs=3  Mode=Multidimensional array  ConcatenateDimension=2
  Mux : Mux  Inputs=3
  Mux1 : Mux  Inputs=3
  Mux2 : Mux  Inputs=3
  "[x]" : Outport
  wires:
  Mux1/1 -> Matrix Concatenate/2
  Mux/1 -> Matrix Concatenate/1
  Mux2/1 -> Matrix Concatenate/3
  Matrix Concatenate/1 -> "[x]"/1
  Gain/1 -> Mux/3
  Gain1/1 -> Mux1/1
  Gain2/1 -> Mux2/2
  Constant/1 -> Mux/1, Mux1/2, Mux2/3
  x/1 -> Demux/1
  Demux/3 -> Gain1/1, Mux/2  "z"
  Demux/2 -> Mux2/1, Gain/1  "y"
  Demux/1 -> Gain2/1, Mux1/3  "x"

== system moto/Subsystem3/axisAngleToRotMat/vec2skew ==
  x : Inport
  Constant : Constant  Value=0
  Demux : Demux  Outputs=3
  Gain : Gain  Gain=-1
  Gain1 : Gain  Gain=-1
  Gain2 : Gain  Gain=-1
  Matrix Concatenate : Concatenate  NumInputs=3  Mode=Multidimensional array  ConcatenateDimension=2
  Mux : Mux  Inputs=3
  Mux1 : Mux  Inputs=3
  Mux2 : Mux  Inputs=3
  "[x]" : Outport
  wires:
  Mux1/1 -> Matrix Concatenate/2
  Mux/1 -> Matrix Concatenate/1
  Mux2/1 -> Matrix Concatenate/3
  Matrix Concatenate/1 -> "[x]"/1
  Gain/1 -> Mux/3
  Gain1/1 -> Mux1/1
  Gain2/1 -> Mux2/2
  Constant/1 -> Mux/1, Mux1/2, Mux2/3
  x/1 -> Demux/1
  Demux/3 -> Gain1/1, Mux/2  "z"
  Demux/2 -> Mux2/1, Gain/1  "y"
  Demux/1 -> Gain2/1, Mux1/3  "x"

== system moto/Subsystem3/screwDistanceToPos/vec2skew ==
  x : Inport
  Constant : Constant  Value=0
  Demux : Demux  Outputs=3
  Gain : Gain  Gain=-1
  Gain1 : Gain  Gain=-1
  Gain2 : Gain  Gain=-1
  Matrix Concatenate : Concatenate  NumInputs=3  Mode=Multidimensional array  ConcatenateDimension=2
  Mux : Mux  Inputs=3
  Mux1 : Mux  Inputs=3
  Mux2 : Mux  Inputs=3
  "[x]" : Outport
  wires:
  Mux1/1 -> Matrix Concatenate/2
  Mux/1 -> Matrix Concatenate/1
  Mux2/1 -> Matrix Concatenate/3
  Matrix Concatenate/1 -> "[x]"/1
  Gain/1 -> Mux/3
  Gain1/1 -> Mux1/1
  Gain2/1 -> Mux2/2
  Constant/1 -> Mux/1, Mux1/2, Mux2/3
  x/1 -> Demux/1
  Demux/3 -> Gain1/1, Mux/2  "z"
  Demux/2 -> Mux2/1, Gain/1  "y"
  Demux/1 -> Gain2/1, Mux1/3  "x"

== system moto/Subsystem4/axisAngleToRotMat/vec2skew ==
  x : Inport
  Constant : Constant  Value=0
  Demux : Demux  Outputs=3
  Gain : Gain  Gain=-1
  Gain1 : Gain  Gain=-1
  Gain2 : Gain  Gain=-1
  Matrix Concatenate : Concatenate  NumInputs=3  Mode=Multidimensional array  ConcatenateDimension=2
  Mux : Mux  Inputs=3
  Mux1 : Mux  Inputs=3
  Mux2 : Mux  Inputs=3
  "[x]" : Outport
  wires:
  Mux1/1 -> Matrix Concatenate/2
  Mux/1 -> Matrix Concatenate/1
  Mux2/1 -> Matrix Concatenate/3
  Matrix Concatenate/1 -> "[x]"/1
  Gain/1 -> Mux/3
  Gain1/1 -> Mux1/1
  Gain2/1 -> Mux2/2
  Constant/1 -> Mux/1, Mux1/2, Mux2/3
  x/1 -> Demux/1
  Demux/3 -> Gain1/1, Mux/2  "z"
  Demux/2 -> Mux2/1, Gain/1  "y"
  Demux/1 -> Gain2/1, Mux1/3  "x"

== system moto/Subsystem4/screwDistanceToPos/vec2skew ==
  x : Inport
  Constant : Constant  Value=0
  Demux : Demux  Outputs=3
  Gain : Gain  Gain=-1
  Gain1 : Gain  Gain=-1
  Gain2 : Gain  Gain=-1
  Matrix Concatenate : Concatenate  NumInputs=3  Mode=Multidimensional array  ConcatenateDimension=2
  Mux : Mux  Inputs=3
  Mux1 : Mux  Inputs=3
  Mux2 : Mux  Inputs=3
  "[x]" : Outport
  wires:
  Mux1/1 -> Matrix Concatenate/2
  Mux/1 -> Matrix Concatenate/1
  Mux2/1 -> Matrix Concatenate/3
  Matrix Concatenate/1 -> "[x]"/1
  Gain/1 -> Mux/3
  Gain1/1 -> Mux1/1
  Gain2/1 -> Mux2/2
  Constant/1 -> Mux/1, Mux1/2, Mux2/3
  x/1 -> Demux/1
  Demux/3 -> Gain1/1, Mux/2  "z"
  Demux/2 -> Mux2/1, Gain/1  "y"
  Demux/1 -> Gain2/1, Mux1/3  "x"
